simulink model "testGauges"  (R2020b)
settings: Solver=VariableStepAuto  StartTime=0.0  StopTime=10.0  RelTol=1e-3
settings Model: EnablePacing=on  VariantFading=off  Creator=grouleau  LastModifiedBy=guy

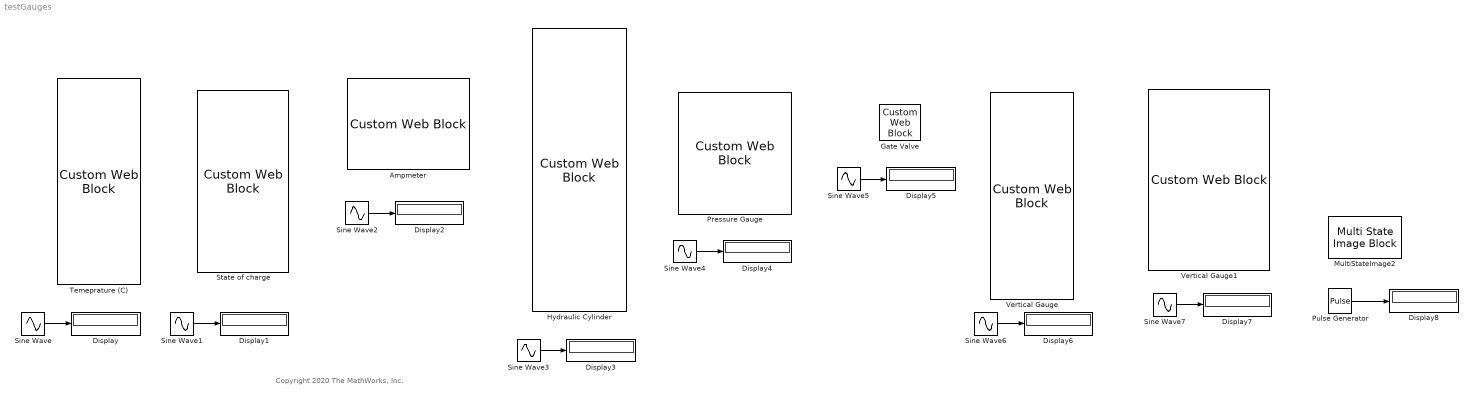
== system testGauges ==
  note: Copyright 2020 The MathWorks, Inc.
  Ampmeter : CustomWebBlock  LabelPosition=Hide  Configuration="{\"components\":[{\"name\":\"CircularScaleComponent\",\"settings\":{\"bounds\":{\"max\":12,\"min\":-12,\"tickInterval\":23.9999999999999},\"direction\":\"cw\",\"flipLimits\":0,\"innerRadius\":0.75,\"internalTickHeightScaleFactor\":1,\"labelColor\":[38,38,38],\"labelFont\":{\"font\":\"Arial\",\"fontSize\":12},\"labelTransparency\":0,\"minorTickHeightScaleFactor\":0.2,\"needleImage\":{\"size\":[96,288],\"src\":\"data:image\\/svg+xml;base64,PHN2ZyB3aWR0aD0iOTYiIGhlaWdodD0iMjg4IiB4bWxucz0iaHR0cDovL3d3dy53My5vcmcvMjAwMC9zdmciIHhtbG5zOnhsaW5rPSJodHRwOi8vd3d3LnczLm9yZy8xOTk5L3hsaW5rIiBvdmVyZmxvdz0iaGlkZGVuIj48ZGVmcz48Y2xpcFBhdGggaWQ9ImNsaXAwIj48cGF0aCBkPSJNMCAwIDk2IDAgOTYgMjg4IDAgMjg4WiIgZmlsbC1ydWxlPSJldmVub2RkIiBjbGlwLXJ1bGU9ImV2ZW5vZGQiLz48L2NsaXBQYXRoPjwvZGVmcz48ZyBjbGlwLXBhdGg9InVybCgjY2xpcDApIj48cmVjdCB4PSIwIiB5PSIwIiB3aWR0aD0iOTYiIGhlaWdodD0iMjg4IiBmaWxsPSIjRkZGRkZGIiBmaWxsLW9wYWNpdHk9IjAiLz48cGF0aCBkPSJNNDguNTAwMSA0MS41MDAxIDQ4LjUwMDIgMjQ3LjUiIHN0cm9rZT0iIzAwMDAwMCIgc3Ryb2tlLXdpZHRoPSI3IiBzdHJva2UtbGluZWNhcD0icm91bmQiIHN0cm9rZS1taXRlcmxpbWl0PSI4IiBmaWxsPSJub25lIiBmaWxsLXJ1bGU9ImV2ZW5vZGQiLz48L2c+PC9zdmc+\"},\"needleOffset\":[0.09442302068368028,0],\"needleOrientation\":-45,\"needleRotation\":90,\"needleSize\":{\"height\":0.36796446559573437,\"width\":0.26380868795837903},\"outerRadius\":0.9,\"position\":[0.17317708333333334,0.05625,0.891796875,0.7701822916666666],\"scaleAngle\":145.25613527122786,\"scaleAngleOffset\":197.0817568691423,\"scaleColors\":[],\"scaleColorsSize\":0.2,\"scalePosition\":[0,0,1,1],\"showLabels\":1,\"showMinorTicks\":1,\"showSpanLine\":1,\"showTicks\":1,\"tickColor\":[0,0,0],\"tickTransparency\":1,\"valueBarColor\":[0,114,189],\"valueBarPosition\":[0,0,1,1],\"valueBarSize\":0.2,\"valueBarTransparency\":0}},{\"name\":\"BackgroundImageComponent\",\"settings\":{\"image\":{\"size\":[384,288],\"src\":\"data:image\\/svg+xml;base64,PHN2ZyB3aWR0aD0iMzg0IiBoZWlnaHQ9IjI4OCIgeG1sbnM9Imh0dHA6Ly93d3cudzMub3JnLzIwMDAvc3ZnIiB4bWxuczp4bGluaz0iaHR0cDovL3d3dy53My5vcmcvMTk5OS94bGluayIgb3ZlcmZsb3c9ImhpZGRlbiI+PGRlZnM+PGNsaXBQYXRoIGlkPSJjbGlwMCI+PHBhdGggZD0iTTAgMCAzODQgMCAzODQgMjg4IDAgMjg4WiIgZmlsbC1ydWxlPSJldmVub2RkIiBjbGlwLXJ1bGU9ImV2ZW5vZGQiLz48L2NsaXBQYXRoPjwvZGVmcz48ZyBjbGlwLXBhdGg9InVybCgjY2xpcDApIj48cmVjdCB4PSIwIiB5PSIwIiB3aWR0aD0iMzg0IiBoZWlnaHQ9IjI4OCIgZmlsbD0iI0ZGRkZGRiIvPjxwYXRoIGQ9Ik0yNy41MDAxIDYxLjgzNDJDMjcuNTAwMSAzOS4wMDYgNDYuMDA2IDIwLjUwMDEgNjguODM0MSAyMC41MDAxTDMxNi4xNjYgMjAuNTAwMUMzMzguOTk0IDIwLjUwMDEgMzU3LjUgMzkuMDA2IDM1Ny41IDYxLjgzNDJMMzU3LjUgMjI3LjE2NkMzNTcuNSAyNDkuOTk0IDMzOC45OTQgMjY4LjUgMzE2LjE2NiAyNjguNUw2OC44MzQxIDI2OC41QzQ2LjAwNiAyNjguNSAyNy41MDAxIDI0OS45OTQgMjcuNTAwMSAyMjcuMTY2WiIgc3Ryb2tlPSIjMDAwMDAwIiBzdHJva2Utd2lkdGg9IjciIHN0cm9rZS1taXRlcmxpbWl0PSI4IiBmaWxsPSJub25lIiBmaWxsLXJ1bGU9ImV2ZW5vZGQiLz48dGV4dCBmb250LWZhbWlseT0iQXJpYWwgUm91bmRlZCBNVCxBcmlhbCBSb3VuZGVkIE1UX01TRm9udFNlcnZpY2Usc2Fucy1zZXJpZiIgZm9udC13ZWlnaHQ9IjcwMCIgZm9udC1zaXplPSI3MiIgdHJhbnNmb3JtPSJ0cmFuc2xhdGUoMTY1LjU4MyAyNTQpIj5BPC90ZXh0PjxwYXRoIGQ9Ik00OS41MDAxIDY2LjY2NzFDNDkuNTAwMSA1My4zMiA2MC4zMiA0Mi41MDAxIDczLjY2NzEgNDIuNTAwMUwzMTEuMzMzIDQyLjUwMDFDMzI0LjY4IDQyLjUwMDEgMzM1LjUgNTMuMzIgMzM1LjUgNjYuNjY3MUwzMzUuNSAxNjMuMzMzQzMzNS41IDE3Ni42OCAzMjQuNjggMTg3LjUgMzExLjMzMyAxODcuNUw3My42NjcxIDE4Ny41QzYwLjMyIDE4Ny41IDQ5LjUwMDEgMTc2LjY4IDQ5LjUwMDEgMTYzLjMzM1oiIHN0cm9rZT0iIzAwMDAwMCIgc3Ryb2tlLXdpZHRoPSI3IiBzdHJva2UtbWl0ZXJsaW1pdD0iOCIgZmlsbD0ibm9uZSIgZmlsbC1ydWxlPSJldmVub2RkIi8+PHBhdGggZD0iTTE1My41IDE4N0MxNTMuNSAxNjUuNzM3IDE3MC43MzcgMTQ4LjUgMTkyIDE0OC41IDIxMy4yNjMgMTQ4LjUgMjMwLjUgMTY1LjczNyAyMzAuNSAxODcgMjMwLjUgMTg3LjExNSAyMzAuNSAxODcuMjMgMjMwLjQ5OCAxODcuMzQ2TDE5MiAxODdaIiBzdHJva2U9IiMwMDAwMDAiIHN0cm9rZS13aWR0aD0iNyIgc3Ryb2tlLW1pdGVybGltaXQ9IjgiIGZpbGw9Im5vbmUiIGZpbGwtcnVsZT0iZXZlbm9kZCIvPjwvZz48L3N2Zz4=\",\"srcOrientation\":\"horizontal\"},\"position\":[0,0,1,1],\"scaleMode\":\"0\"}},{\"name\":\"ForegroundImageComponent\",\"settings\":{\"image\":{\"size\":[0,0],\"src\":\"default\",\"srcOrientation\":[]},\"isForeground\":1,\"position\":[0,0,1,1],\"scaleMode\":\"0\"}}],\"settings\":{\"BindingType\":\"signal\",\"aspectRatio\":1.3333333333333333,\"direction\":\"cw\",\"fixedAspectRatio\":\"on\",\"flipLimits\":0,\"orientation\":\"horizontal\",\"value\":-12},\"type\":\"CircularGauge\"}"
  Display{,1..8} (9 alike) : Display
  Gate Valve : CustomWebBlock  LabelPosition=Hide  Configuration="{\"components\":[{\"name\":\"LinearScaleComponent\",\"settings\":{\"bounds\":{\"max\":1,\"min\":0,\"tickInterval\":\"auto\"},\"internalTickHeightScaleFactor\":0.5,\"labelColor\":[250,245,199],\"labelFont\":{\"font\":\"Arial\",\"fontSize\":12},\"labelTransparency\":0,\"needleImage\":{\"size\":[0,0],\"src\":\"\",\"srcOrientation\":\"vertical\"},\"needleOffset\":[0,0],\"needleSize\":{\"height\":0,\"width\":0},\"position\":[0.036458333333333336,0.0695754716981132,3.4033018867924527,0.919921875],\"scaleColors\":[],\"scaleColorsSize\":0.2,\"showLabels\":1,\"showMinorTicks\":0,\"showSpanLine\":1,\"showTicks\":1,\"tickColor\":[250,245,200],\"tickTransparency\":0,\"valueBarColor\":[0,0,0],\"valueBarOffset\":0,\"valueBarSize\":0.23,\"valueBarTransparency\":1}},{\"name\":\"BackgroundImageComponent\",\"settings\":{\"image\":{\"size\":[0,0],\"src\":\"default\",\"srcOrientation\":null},\"position\":[0,0,1,1],\"scaleMode\":\"0\"}},{\"name\":\"ForegroundImageComponent\",\"settings\":{\"image\":{\"size\":[53,48],\"src\":\"data:image\\/png;base64,iVBORw0KGgoAAAANSUhEUgAAAp0AAAJbCAYAAACmZC+XAAAACXBIWXMAAA7EAAAOxAGVKw4bAAAAB3RJTUUH5AoDETghXxYhmQAAIABJREFUeJzs3XtwVeW9\\/\\/HPLqBEKwRNuA3BpAoElJsBArEmgtwsRUkEWqiECug0iMgPM8Fr05wZR0+agwoRLEoqwRJFIKnIMQGEBksgQORmuWMiMFwEJWBruMX1+4OSAzZr7Z2w98rea79fM4xOnmctvtOa\\/Xz291kXl2EYhgAAAAAf+klDFwAAAADnI3QCAADA5widAAAA8DlCJwAAAHyO0AkAAACfI3QCAADA5widAAAA8DlCJwAAAHyu8fUc7HK5vFUHAAAAAkR93i1EpxMAAAA+R+gEAACAzx ...(+27118 chars)\",\"srcOrientation\":\"vertical\"},\"isForeground\":1,\"position\":[0,0,1,1],\"scaleMode\":\"0\"}}],\"settings\":{\"BindingType\":\"signal\",\"aspectRatio\":0.2647058823529412,\"fixedAspectRatio\":\"off\",\"orientation\":\"vertical\",\"value\":0},\"type\":\"LinearGauge\"}"
  Hydraulic Cylinder : CustomWebBlock  LabelPosition=Hide  Configuration="{\"components\":[{\"name\":\"LinearScaleComponent\",\"settings\":{\"bounds\":{\"max\":12,\"min\":0,\"tickInterval\":\"auto\"},\"internalTickHeightScaleFactor\":0.5,\"labelColor\":[250,245,199],\"labelFont\":{\"font\":\"Arial\",\"fontSize\":12},\"labelTransparency\":0,\"needleImage\":{\"size\":[192,576],\"src\":\"data:image\\/svg+xml;base64,PHN2ZyB3aWR0aD0iMTkyIiBoZWlnaHQ9IjU3NiIgeG1sbnM9Imh0dHA6Ly93d3cudzMub3JnLzIwMDAvc3ZnIiB4bWxuczp4bGluaz0iaHR0cDovL3d3dy53My5vcmcvMTk5OS94bGluayIgb3ZlcmZsb3c9ImhpZGRlbiI+PGRlZnM+PGNsaXBQYXRoIGlkPSJjbGlwMCI+PHBhdGggZD0iTTAgMCAxOTIgMCAxOTIgNTc2IDAgNTc2WiIgZmlsbC1ydWxlPSJldmVub2RkIiBjbGlwLXJ1bGU9ImV2ZW5vZGQiLz48L2NsaXBQYXRoPjwvZGVmcz48ZyBjbGlwLXBhdGg9InVybCgjY2xpcDApIj48cmVjdCB4PSIwIiB5PSIwIiB3aWR0aD0iMTkyIiBoZWlnaHQ9IjU3NiIgZmlsbD0iI0ZGRkZGRiIgZmlsbC1vcGFjaXR5PSIwIi8+PHJlY3QgeD0iNzkuNTAwMSIgeT0iMTIxLjUiIHdpZHRoPSIzMiIgaGVpZ2h0PSI0NTIiIHN0cm9rZT0iIzAwMDAwMCIgc3Ryb2tlLXdpZHRoPSI3IiBzdHJva2UtbWl0ZXJsaW1pdD0iOCIgZmlsbD0iI0E2QTZBNiIvPjxwYXRoIGQ9Ik00MC41MDAxIDU4QzQwLjUwMDEgMjcuOTAwNSA2NC45MDA1IDMuNTAwMDUgOTUgMy41MDAwNSAxMjUuMSAzLjUwMDA1IDE0OS41IDI3LjkwMDUgMTQ5LjUgNTggMTQ5LjUgODguMDk5NiAxMjUuMSAxMTIuNSA5NSAxMTIuNSA2NC45MDA1IDExMi41IDQwLjUwMDEgODguMDk5NiA0MC41MDAxIDU4WiIgc3Ryb2tlPSIjMDAwMDAwIiBzdHJva2Utd2lkdGg9IjUiIHN0cm9rZS1taXRlcmxpbWl0PSI4IiBmaWxsPSIjNDQ3MkM0IiBmaWxsLXJ1bGU9ImV2ZW5vZGQiLz48cmVjdCB4PSI2MS41MDAxIiB5PSIxMDEuNSIgd2lkdGg9IjY5IiBoZWlnaHQ9IjIwIiBzdHJva2U9IiMwMDAwMDAiIHN0cm9rZS13aWR0aD0iNyIgc3Ryb2tlLW1pdGVybGltaXQ9IjgiIGZpbGw9IiM0NDcyQzQiLz48cGF0aCBkPSJNNjQuNTAwMSA1NS4wMDAxQzY0LjUwMDEgMzguMTU1NCA3OC4xNTU0IDI0LjUwMDEgOTUuMDAwMSAyNC41MDAxIDExMS44NDUgMjQuNTAwMSAxMjUuNSAzOC4xNTU0IDEyNS41IDU1LjAwMDEgMTI1LjUgNzEuODQ0NyAxMTEuODQ1IDg1LjUwMDEgOTUuMDAwMSA4NS41MDAxIDc4LjE1NTQgODUuNTAwMSA2NC41MDAxIDcxLjg0NDcgNjQuNTAwMSA1NS4wMDAxWiIgc3Ryb2tlPSIjMDAwMDAwIiBzdHJva2Utd2lkdGg9IjUiIHN0cm9rZS1taXRlcmxpbWl0PSI4IiBmaWxsPSIjRkZGRkZGIiBmaWxsLXJ1bGU9ImV2ZW5vZGQiLz48L2c+PC9zdmc+\",\"srcOrientation\":\"vertical\"},\"needleOffset\":[0.1248509420462676,-0.19590382902938558],\"needleSize\":{\"height\":0.5599626068376068,\"width\":0.5998931623931624},\"position\":[0.2412014563106796,0.2516084558823529,0.5994944852941176,0.39638956310679613],\"scaleColors\":[],\"scaleColorsSize\":0.2,\"showLabels\":1,\"showMinorTicks\":0,\"showSpanLine\":1,\"showTicks\":1,\"tickColor\":[250,245,200],\"tickTransparency\":0,\"valueBarColor\":[23,89,176],\"valueBarOffset\":0,\"valueBarSize\":0.23,\"valueBarTransparency\":0}},{\"name\":\"BackgroundImageComponent\",\"settings\":{\"image\":{\"size\":[0,0],\"src\":\"default\",\"srcOrientation\":null},\"position\":[0,0,1,1],\"scaleMode\":\"0\"}},{\"name\":\"ForegroundImageComponent\",\"settings\":{\"image\":{\"size\":[288,1056],\"src\":\"data:image\\/svg+xml;base64,PHN2ZyB3aWR0aD0iMjg4IiBoZWlnaHQ9IjEwNTYiIHhtbG5zPSJodHRwOi8vd3d3LnczLm9yZy8yMDAwL3N2ZyIgeG1sbnM6eGxpbms9Imh0dHA6Ly93d3cudzMub3JnLzE5OTkveGxpbmsiIG92ZXJmbG93PSJoaWRkZW4iPjxkZWZzPjxjbGlwUGF0aCBpZD0iY2xpcDAiPjxwYXRoIGQ9Ik0wIDAgMjg4IDAgMjg4IDEwNTYgMCAxMDU2WiIgZmlsbC1ydWxlPSJldmVub2RkIiBjbGlwLXJ1bGU9ImV2ZW5vZGQiLz48L2NsaXBQYXRoPjwvZGVmcz48ZyBjbGlwLXBhdGg9InVybCgjY2xpcDApIj48cmVjdCB4PSIwIiB5PSIwIiB3aWR0aD0iMjg4IiBoZWlnaHQ9IjEwNTYiIGZpbGw9IiNGRkZGRkYiIGZpbGwtb3BhY2l0eT0iMCIvPjxyZWN0IHg9Ijg1LjUwMDEiIHk9IjYzMC41IiB3aWR0aD0iMTE1IiBoZWlnaHQ9IjM2NyIgc3Ryb2tlPSIjMDAwMDAwIiBzdHJva2Utd2lkdGg9IjciIHN0cm9rZS1taXRlcmxpbWl0PSI4IiBmaWxsPSIjNDQ3MkM0Ii8+PHJlY3QgeD0iNzEuNTAwMSIgeT0iNTgxLjUiIHdpZHRoPSIxNDYiIGhlaWdodD0iNDkiIHN0cm9rZT0iIzAwMDAwMCIgc3Ryb2tlLXdpZHRoPSI3IiBzdHJva2UtbWl0ZXJsaW1pdD0iOCIgZmlsbD0iIzQ0NzJDNCIvPjxwYXRoIGQ9Ik0yMDAuNSA5ODkuNUMyMDAuNSAxMDIxLjUzIDE3NC43NTYgMTA0Ny41IDE0MyAxMDQ3LjUgMTExLjQ5IDEwNDcuNSA4NS44NTAyIDEwMjEuOTIgODUuNTAzNCA5OTAuMTM4TDE0MyA5ODkuNVoiIHN0cm9rZT0iIzAwMDAwMCIgc3Ryb2tlLXdpZHRoPSI3IiBzdHJva2UtbWl0ZXJsaW1pdD0iOCIgZmlsbD0iIzQ0NzJDNCIgZmlsbC1ydWxlPSJldmVub2RkIi8+PHJlY3QgeD0iOTAiIHk9Ijk0NSIgd2lkdGg9IjEwOCIgaGVpZ2h0PSI0OSIgZmlsbD0iIzQ0NzJDNCIvPjxwYXRoIGQ9Ik0xMDguNSA5ODkuNUMxMDguNSA5NjkuNjE4IDEyNC42MTggOTUzLjUgMTQ0LjUgOTUzLjUgMTY0LjM4MiA5NTMuNSAxODAuNSA5NjkuNjE4IDE4MC41IDk4OS41IDE4MC41IDEwMDkuMzggMTY0LjM4MiAxMDI1LjUgMTQ0LjUgMTAyNS41IDEyNC42MTggMTAyNS41IDEwOC41IDEwMDkuMzggMTA4LjUgOTg5LjVaIiBzdHJva2U9IiMwMDAwMDAiIHN0cm9rZS13aWR0aD0iNSIgc3Ryb2tlLW1pdGVybGltaXQ9IjgiIGZpbGw9IiNGRkZGRkYiIGZpbGwtcnVsZT0iZXZlbm9kZCIvPjwvZz48L3N2Zz4=\",\"srcOrientation\":\"vertical\"},\"isForeground\":1,\"position\":[0,0,1,1],\"scaleMode\":\"0\"}}],\"settings\":{\"BindingType\":\"signal\",\"aspectRatio\":0.3333333333333333,\"fixedAspectRatio\":\"on\",\"orientation\":\"vertical\",\"value\":0},\"type\":\"LinearGauge\"}"
  MultiStateImage2 : MultiStateImageBlock  LabelPosition=Hide
  Pressure Gauge : CustomWebBlock  LabelPosition=Hide  Configuration="{\"components\":[{\"name\":\"CircularScaleComponent\",\"settings\":{\"bounds\":{\"max\":2500,\"min\":0,\"tickInterval\":\"auto\"},\"direction\":\"cw\",\"flipLimits\":0,\"innerRadius\":0.75,\"internalTickHeightScaleFactor\":1,\"labelColor\":[38,38,38],\"labelFont\":{\"font\":\"Arial\",\"fontSize\":12},\"labelTransparency\":1,\"minorTickHeightScaleFactor\":0.2,\"needleImage\":{\"size\":[79,20],\"src\":\"data:image\\/svg+xml;base64,PD94bWwgdmVyc2lvbj0iMS4wIiBlbmNvZGluZz0idXRmLTgiPz4KPCEtLSBHZW5lcmF0b3I6IEFkb2JlIElsbHVzdHJhdG9yIDI0LjEuMiwgU1ZHIEV4cG9ydCBQbHVnLUluIC4gU1ZHIFZlcnNpb246IDYuMDAgQnVpbGQgMCkgIC0tPgo8c3ZnIHZlcnNpb249IjEuMSIgaWQ9IkxheWVyXzEiIHhtbG5zPSJodHRwOi8vd3d3LnczLm9yZy8yMDAwL3N2ZyIgeG1sbnM6eGxpbms9Imh0dHA6Ly93d3cudzMub3JnLzE5OTkveGxpbmsiIHg9IjBweCIgeT0iMHB4IgoJIHZpZXdCb3g9IjAgMCA3OC43IDIwIiBzdHlsZT0iZW5hYmxlLWJhY2tncm91bmQ6bmV3IDAgMCA3OC43IDIwOyIgeG1sOnNwYWNlPSJwcmVzZXJ2ZSI+CjxwYXRoIGQ9Ik01My4xLDUuOGwyNS42LTEuNGwtMy41LDVsMy4xLDUuMmwtMjUuNC0xLjNjLTEuNSwyLjMtNC4yLDMuNC02LjksM2MtMi4yLTAuMy00LjItMS43LTUuMi0zLjdMMC45LDEwLjgKCWMtMS4xLDAtMS4yLTEuNi0wLjEtMS43bDM5LjktMi43QzQyLDMuNiw0NSwyLDQ4LDIuNEM1MC4yLDIuOCw1Miw0LDUzLjEsNS44TDUzLjEsNS44eiBNNTMuNywxMS42bDIxLjQsMS4xbC0yLTMuNGwyLjEtMy4xCglMNTMuOCw3LjVDNTMuOSw4LDU0LDguNSw1NCw5LjFDNTQuMSw5LjksNTQsMTAuOCw1My43LDExLjZMNTMuNywxMS42eiBNNDAuMSw4LjJMMTkuMyw5LjVjLTMuOSwwLjMtMy45LDAuMiwwLDAuNGwyMC45LDEKCUM0MCwxMC41LDQwLDEwLDQwLDkuNUM0MCw5LjEsNDAsOC42LDQwLjEsOC4yTDQwLjEsOC4yeiBNNDcuOCw0LjFjLTMuMy0wLjUtNi4yLDIuMS02LjEsNS40YzAsMi42LDEuOSw0LjgsNC41LDUuMQoJYzMuMywwLjUsNi4zLTIuMiw2LjEtNS41QzUyLjIsNi42LDUwLjMsNC41LDQ3LjgsNC4xTDQ3LjgsNC4xeiIvPgo8L3N2Zz4K\"},\"needleOffset\":[0.061149395709068396,0],\"needleOrientation\":-45,\"needleRotation\":180,\"needleSize\":{\"height\":0.1101177838554453,\"width\":0.43719941652583294},\"outerRadius\":0.9,\"position\":[0.0065,0.1379808323486937,0.7195746356833399,0.726],\"scaleAngle\":270,\"scaleAngleOffset\":135,\"scaleColors\":[],\"scaleColorsSize\":0.2,\"scalePosition\":[0,0,1,1],\"showLabels\":1,\"showMinorTicks\":1,\"showSpanLine\":1,\"showTicks\":1,\"tickColor\":[38,38,38],\"tickTransparency\":1,\"valueBarColor\":[0,114,189],\"valueBarPosition\":[0,0,1,1],\"valueBarSize\":0.2,\"valueBarTransparency\":0}},{\"name\":\"BackgroundImageComponent\",\"settings\":{\"image\":{\"size\":[6248,6456],\"src\":\"data:image\\/svg+xml;base64,PD94bWwgdmVyc2lvbj0iMS4wIiBlbmNvZGluZz0idXRmLTgiPz4KPCEtLSBHZW5lcmF0b3I6IEFkb2JlIElsbHVzdHJhdG9yIDI0LjEuMiwgU1ZHIEV4cG9ydCBQbHVnLUluIC4gU1ZHIFZlcnNpb246IDYuMDAgQnVpbGQgMCkgIC0tPgo8c3ZnIHZlcnNpb249IjEuMSIgaWQ9IkxheWVyXzEiIHhtbG5zOnhvZG09Imh0dHA6Ly93d3cuY29yZWwuY29tL2NvcmVsZHJhdy9vZG0vMjAwMyIKCSB4bWxucz0iaHR0cDovL3d3dy53My5vcmcvMjAwMC9zdmciIHhtbG5zOnhsaW5rPSJodHRwOi8vd3d3LnczLm9yZy8xOTk5L3hsaW5rIiB4 ...(+3504 chars)\",\"srcOrientation\":\"horizontal\"},\"position\":[0,0,1,1],\"scaleMode\":\"0\"}},{\"name\":\"ForegroundImageComponent\",\"settings\":{\"image\":{\"size\":[0,0],\"src\":\"default\",\"srcOrientation\":[]},\"isForeground\":1,\"position\":[0,0,1,1],\"scaleMode\":\"0\"}}],\"settings\":{\"BindingType\":\"signal\",\"aspectRatio\":0.9677819083023544,\"direction\":\"cw\",\"fixedAspectRatio\":\"on\",\"flipLimits\":0,\"orientation\":\"horizontal\",\"value\":0},\"type\":\"CircularGauge\"}"
  Pulse Generator : DiscretePulseGenerator  PulseType=Time based  Period=4  PulseWidth=50
  Sine Wave : Sin  Amplitude=25  Bias=25  SampleTime=0
  Sine Wave1 : Sin  Amplitude=0.5  Bias=0.5  SampleTime=0
  Sine Wave2 : Sin  Amplitude=12  SampleTime=0
  Sine Wave3 : Sin  Amplitude=6  Bias=6  SampleTime=0
  Sine Wave4 : Sin  Amplitude=2500/2  Bias=2500/2  SampleTime=0
  Sine Wave5 : Sin  Amplitude=0.5  Bias=0.5  SampleTime=0
  Sine Wave6 : Sin  Amplitude=12.5  Bias=12.5  SampleTime=0
  Sine Wave7 : Sin  Amplitude=50  Bias=50  SampleTime=0
  State of charge : CustomWebBlock  LabelPosition=Hide  Configuration="{\"components\":[{\"name\":\"LinearScaleComponent\",\"settings\":{\"bounds\":{\"max\":1,\"min\":0,\"tickInterval\":0.2},\"internalTickHeightScaleFactor\":0.5,\"labelColor\":[0,0,0],\"labelFont\":{\"font\":\"Arial\",\"fontSize\":12},\"labelTransparency\":0,\"needleImage\":{\"size\":[0,0],\"src\":\"\",\"srcOrientation\":\"vertical\"},\"needleOffset\":[0,0],\"needleSize\":{\"height\":0,\"width\":0},\"position\":[0.0662421218487395,0.10333508403361344,2.7942489495798317,0.9641544117647058],\"scaleColors\":[],\"scaleColorsSize\":0.2,\"showLabels\":1,\"showMinorTicks\":0,\"showSpanLine\":1,\"showTicks\":1,\"tickColor\":[38,38,38],\"tickTransparency\":0,\"valueBarColor\":[23,89,176],\"valueBarOffset\":0,\"valueBarSize\":0.23,\"valueBarTransparency\":1}},{\"name\":\"BackgroundImageComponent\",\"settings\":{\"image\":{\"size\":[192,384],\"src\":\"data:image\\/svg+xml;base64,PHN2ZyB3aWR0aD0iMTkyIiBoZWlnaHQ9IjM4NCIgeG1sbnM9Imh0dHA6Ly93d3cudzMub3JnLzIwMDAvc3ZnIiB4bWxuczp4bGluaz0iaHR0cDovL3d3dy53My5vcmcvMTk5OS94bGluayIgb3ZlcmZsb3c9ImhpZGRlbiI+PGRlZnM+PGNsaXBQYXRoIGlkPSJjbGlwMCI+PHBhdGggZD0iTTAgMCAxOTIgMCAxOTIgMzg0IDAgMzg0WiIgZmlsbC1ydWxlPSJldmVub2RkIiBjbGlwLXJ1bGU9ImV2ZW5vZGQiLz48L2NsaXBQYXRoPjwvZGVmcz48ZyBjbGlwLXBhdGg9InVybCgjY2xpcDApIj48cmVjdCB4PSIwIiB5PSIwIiB3aWR0aD0iMTkyIiBoZWlnaHQ9IjM4NCIgZmlsbD0iI0ZGRkZGRiIvPjxwYXRoIGQ9Ik0yMi41MDAxIDU4LjUwMDVDMjIuNTAwMSA0NC42OTMxIDMzLjY5MzEgMzMuNTAwMSA0Ny41MDA1IDMzLjUwMDFMMTQ3LjUgMzMuNTAwMUMxNjEuMzA3IDMzLjUwMDEgMTcyLjUgNDQuNjkzMSAxNzIuNSA1OC41MDA1TDE3Mi41IDM1My41QzE3Mi41IDM2Ny4zMDcgMTYxLjMwNyAzNzguNSAxNDcuNSAzNzguNUw0Ny41MDA1IDM3OC41QzMzLjY5MzEgMzc4LjUgMjIuNTAwMSAzNjcuMzA3IDIyLjUwMDEgMzUzLjVaIiBzdHJva2U9IiMwMDAwMDAiIHN0cm9rZS13aWR0aD0iNyIgc3Ryb2tlLW1pdGVybGltaXQ9IjgiIGZpbGw9Im5vbmUiIGZpbGwtcnVsZT0iZXZlbm9kZCIvPjxwYXRoIGQ9Ik01NiA4LjAwMDA5QzU2IDUuMjM4NjIgNTguMjM4NiAzIDYxLjAwMDEgM0wxMzMgM0MxMzUuNzYxIDMgMTM4IDUuMjM4NjIgMTM4IDguMDAwMDlMMTM4IDI3Ljk5OTlDMTM4IDMwLjc2MTQgMTM1Ljc2MSAzMyAxMzMgMzNMNjEuMDAwMSAzM0M1OC4yMzg2IDMzIDU2IDMwLjc2MTQgNTYgMjcuOTk5OVoiIGZpbGwtcnVsZT0iZXZlbm9kZCIvPjwvZz48L3N2Zz4=\",\"srcOrientation\":\"vertical\"},\"position\":[0,0,1,1],\"scaleMode\":\"0\"}},{\"name\":\"ForegroundImageComponent\",\"settings\":{\"image\":{\"size\":[0,0],\"src\":\"default\",\"srcOrientation\":[]},\"isForeground\":1,\"position\":[0,0,1,1],\"scaleMode\":\"0\"}}],\"settings\":{\"BindingType\":\"signal\",\"aspectRatio\":0.5,\"fixedAspectRatio\":\"on\",\"orientation\":\"vertical\"},\"type\":\"LinearGauge\"}"
  Temeprature (C) : CustomWebBlock  LabelPosition=Hide  Configuration="{\"components\":[{\"name\":\"LinearScaleComponent\",\"settings\":{\"bounds\":{\"max\":50,\"min\":0,\"tickInterval\":\"auto\"},\"internalTickHeightScaleFactor\":0.5,\"labelColor\":[38,38,38],\"labelFont\":{\"font\":\"Arial\",\"fontSize\":12},\"labelTransparency\":1,\"needleImage\":{\"size\":[0,0],\"src\":\"\",\"srcOrientation\":\"vertical\"},\"needleOffset\":[0,0],\"needleSize\":{\"height\":0,\"width\":0},\"position\":[0.06567112546125461,0.0888569374550683,1.3367361610352264,0.692054889298893],\"scaleColors\":[],\"scaleColorsSize\":0.2,\"showLabels\":1,\"showMinorTicks\":0,\"showSpanLine\":1,\"showTicks\":1,\"tickColor\":[0,0,0],\"tickTransparency\":0,\"valueBarColor\":[194,0,0],\"valueBarOffset\":0,\"valueBarSize\":0.23,\"valueBarTransparency\":1}},{\"name\":\"BackgroundImageComponent\",\"settings\":{\"image\":{\"size\":[154,384],\"src\":\"data:image\\/svg+xml;base64,PHN2ZyB3aWR0aD0iMTU0IiBoZWlnaHQ9IjM4NCIgeG1sbnM9Imh0dHA6Ly93d3cudzMub3JnLzIwMDAvc3ZnIiB4bWxuczp4bGluaz0iaHR0cDovL3d3dy53My5vcmcvMTk5OS94bGluayIgb3ZlcmZsb3c9ImhpZGRlbiI+PGRlZnM+PGNsaXBQYXRoIGlkPSJjbGlwMCI+PHBhdGggZD0iTTAgMCAxNTQgMCAxNTQgMzg0IDAgMzg0WiIgZmlsbC1ydWxlPSJldmVub2RkIiBjbGlwLXJ1bGU9ImV2ZW5vZGQiLz48L2NsaXBQYXRoPjwvZGVmcz48ZyBjbGlwLXBhdGg9InVybCgjY2xpcDApIj48cmVjdCB4PSIwIiB5PSIwIiB3aWR0aD0i ...(+1892 chars)\",\"srcOrientation\":\"vertical\"},\"position\":[0,0,1,1],\"scaleMode\":\"0\"}},{\"name\":\"ForegroundImageComponent\",\"settings\":{\"image\":{\"size\":[0,0],\"src\":\"default\",\"srcOrientation\":[]},\"isForeground\":1,\"position\":[0,0,1,1],\"scaleMode\":\"0\"}}],\"settings\":{\"BindingType\":\"signal\",\"aspectRatio\":0.4010416666666667,\"fixedAspectRatio\":\"on\",\"orientation\":\"vertical\"},\"type\":\"LinearGauge\"}"
  Vertical Gauge : CustomWebBlock  LabelPosition=Hide  ShowInitialText=on  Configuration="{\"components\":[{\"name\":\"LinearScaleComponent\",\"settings\":{\"bounds\":{\"max\":25,\"min\":0,\"tickInterval\":\"auto\"},\"internalTickHeightScaleFactor\":1,\"labelColor\":[38,38,38],\"labelFont\":{\"font\":\"Arial\",\"fontSize\":12},\"labelTransparency\":1,\"needleImage\":{\"size\":[298,298],\"src\":\"data:image\\/svg+xml;base64,PHN2ZyB3aWR0aD0iMjk4IiBoZWlnaHQ9IjI5OCIgeG1sbnM9Imh0dHA6Ly93d3cudzMub3JnLzIwMDAvc3ZnIiB4bWxuczp4bGluaz0iaHR0cDovL3d3dy53My5vcmcvMTk5OS94bGluayIgb3ZlcmZsb3c9ImhpZGRlbiI+PGRlZnM+PGNsaXBQYXRoIGlkPSJjbGlwMCI+PHBhdGggZD0iTTAgMCAyOTggMCAyOTggMjk4IDAgMjk4WiIgZmlsbC1ydWxlPSJldmVub2RkIiBjbGlwLXJ1bGU9ImV2ZW5vZGQiLz48L2NsaXBQYXRoPjxyYWRpYWxHcmFkaWVudCBjeD0iMS4wNjU2MWUrMDYiIGN5PSIxLjA2NTYxZSswNiIgcj0iMS41MDdlKzA2IiBmeD0iMS4wNjU2MWUrMDYiIGZ5PSIxLjA2NTYxZSswNiIgZ3JhZGllbnRVbml0cz0idXNlclNwYWNlT25Vc2UiIHNwcmVhZE1ldGhvZD0icGFkIiBpZD0iZmlsbDEiIGdyYWRpZW50VHJhbnNmb3JtPSJtYXRyaXgoMC4wMDAxMDUxMDQgMCAwIDAuMDAwMTA1MTA0IDM3IDQ5KSI+PHN0b3Agb2Zmc2V0PSIwIiBzdG9wLWNvbG9yPSIjQjA1MDBGIi8+PHN0b3Agb2Zmc2V0PSIwLjQ4IiBzdG9wLWNvbG9yPSIjRUU4MTM3Ii8+PHN0b3Agb2Zmc2V0PSIxIiBzdG9wLWNvbG9yPSIjRjRCMTgzIi8+PC9yYWRpYWxHcmFkaWVudD48L2RlZnM+PGcgY2xpcC1wYXRoPSJ1cmwoI2NsaXAwKSI+PHJlY3QgeD0iMCIgeT0iMCIgd2lkdGg9IjI5OCIgaGVpZ2h0PSIyOTgiIGZpbGw9IiNGRkZGRkYiIGZpbGwtb3BhY2l0eT0iMCIvPjxwYXRoIGQ9Ik0zNyAxNjFDMzcgOTkuMTQ0MSA4Ny4xNDQxIDQ5IDE0OSA0OSAyMTAuODU2IDQ5IDI2MSA5OS4xNDQxIDI2MSAxNjEgMjYxIDIyMi44NTYgMjEwLjg1NiAyNzMgMTQ5IDI3MyA4Ny4xNDQxIDI3MyAzNyAyMjIuODU2IDM3IDE2MVoiIHN0cm9rZT0iI0VEN0QzMSIgc3Ryb2tlLXdpZHRoPSIzLjk5OTk2IiBzdHJva2UtbWl0ZXJsaW1pdD0iOCIgZmlsbD0idXJsKCNmaWxsMSkiIGZpbGwtcnVsZT0iZXZlbm9kZCIvPjwvZz48L3N2Zz4=\",\"srcOrientation\":\"vertical\"},\"needleOffset\":[-0.4190231362467866,0.06580976863753213],\"needleSize\":{\"height\":0.22511574074074073,\"width\":0.5627893518518519},\"position\":[0.12858796296296296,0.008391203703703705,1.0219907407407407,0.8446180555555556],\"scaleColors\":[],\"scaleColorsSize\":0.2,\"showLabels\":1,\"showMinorTicks\":0,\"showSpanLine\":false,\"showTicks\":1,\"tickColor\":[166,166,166],\"tickTransparency\":1,\"valueBarColor\":[23,89,176],\"valueBarOffset\":0,\"valueBarSize\":0.23,\"valueBarTransparency\":0}},{\"name\":\"BackgroundImageComponent\",\"settings\":{\"image\":{\"size\":[384,960],\"src\":\"data:image\\/svg+xml;base64,PHN2ZyB3aWR0aD0iMzg0IiBoZWlnaHQ9Ijk2MCIgeG1sbnM9Imh0dHA6Ly93d3cudzMub3JnLzIwMDAvc3ZnIiB4bWxuczp4bGluaz0iaHR0cDovL3d3dy53My5vcmcvMTk5OS94bGluayIgb3ZlcmZsb3c9ImhpZGRlbiI+PGRlZnM+PGNsaXBQYXRoIGlkPSJjbGlwMCI+PHBhdGggZD0iTTAgMCAzODQgMCAzODQgOTYwIDAgOTYwWiIgZmlsbC1ydWxlPSJldmVub2RkIiBjbGlwLXJ1bGU9ImV2ZW5vZGQiLz48L2NsaXBQYXRoPjwvZGVmcz48ZyBjbGlwLXBhdGg9InVybCgjY2xpcDApIj48cmVjdCB4PSIwIiB5PSIwIiB3aWR0aD0i ...(+2956 chars)\",\"srcOrientation\":\"vertical\"},\"position\":[0,0,1,1],\"scaleMode\":\"0\"}},{\"name\":\"ForegroundImageComponent\",\"settings\":{\"image\":{\"size\":[0,0],\"src\":\"default\",\"srcOrientation\":[]},\"isForeground\":1,\"position\":[0,0,1,1],\"scaleMode\":\"0\"}}],\"settings\":{\"BindingType\":\"signal\",\"aspectRatio\":0.4,\"fixedAspectRatio\":\"on\",\"orientation\":\"vertical\",\"value\":0},\"type\":\"LinearGauge\"}"
  Vertical Gauge1 : CustomWebBlock  LabelPosition=Hide  Configuration="{\"components\":[{\"name\":\"LinearScaleComponent\",\"settings\":{\"bounds\":{\"max\":100,\"min\":0,\"tickInterval\":\"auto\"},\"internalTickHeightScaleFactor\":1,\"labelColor\":[38,38,38],\"labelFont\":{\"font\":\"Arial\",\"fontSize\":12},\"labelTransparency\":1,\"needleImage\":{\"size\":[960,384],\"src\":\"data:image\\/svg+xml;base64,PHN2ZyB3aWR0aD0iOTYwIiBoZWlnaHQ9IjM4NCIgeG1sbnM9Imh0dHA6Ly93d3cudzMub3JnLzIwMDAvc3ZnIiB4bWxuczp4bGluaz0iaHR0cDovL3d3dy53My5vcmcvMTk5OS94bGluayIgb3ZlcmZsb3c9ImhpZGRlbiI+PGRlZnM+PGNsaXBQYXRoIGlkPSJjbGlwMCI+PHBhdGggZD0iTTAgMCA5NjAgMCA5NjAgMzg0IDAgMzg0WiIgZmlsbC1ydWxlPSJldmVub2RkIiBjbGlwLXJ1bGU9ImV2ZW5vZGQiLz48L2NsaXBQYXRoPjxpbWFnZSB3aWR0aD0iNzUiIGhlaWdodD0iODQiIHhsaW5rOmhyZWY9ImRhdGE6aW1hZ2UvanBlZzti ...(+118888 chars)\",\"srcOrientation\":\"vertical\"},\"needleOffset\":[-0.3472684876748834,0.002165982672138623],\"needleSize\":{\"height\":0.3941701680672269,\"width\":0.8638960015757337},\"position\":[0.530921743697479,0.04421902698443963,0.818790624384479,0.4299501050420168],\"scaleColors\":[],\"scaleColorsSize\":0.2,\"showLabels\":false,\"showMinorTicks\":0,\"showSpanLine\":false,\"showTicks\":false,\"tickColor\":[38,38,38],\"tickTransparency\":1,\"valueBarColor\":[0,187,205],\"valueBarOffset\":0.02,\"valueBarSize\":1,\"valueBarTransparency\":1}},{\"name\":\"BackgroundImageComponent\",\"settings\":{\"image\":{\"size\":[480,720],\"src\":\"data:image\\/svg+xml;base64,PHN2ZyB3aWR0aD0iNDgwIiBoZWlnaHQ9IjcyMCIgeG1sbnM9Imh0dHA6Ly93d3cudzMub3JnLzIwMDAvc3ZnIiB4bWxuczp4bGluaz0iaHR0cDovL3d3dy53My5vcmcvMTk5OS94bGluayIgb3ZlcmZsb3c9ImhpZGRlbiI+PGRlZnM+PGNsaXBQYXRoIGlkPSJjbGlwMCI+PHBhdGggZD0iTTAgMCA0ODAgMCA0ODAgNzIwIDAgNzIwWiIgZmlsbC1ydWxlPSJldmVub2RkIiBjbGlwLXJ1bGU9ImV2ZW5vZGQiLz48L2NsaXBQYXRoPjwvZGVmcz48ZyBjbGlwLXBhdGg9InVybCgjY2xpcDApIj48cmVjdCB4PSIwIiB5PSIwIiB3aWR0aD0i ...(+1700 chars)\",\"srcOrientation\":\"vertical\"},\"position\":[0,0,1,1],\"scaleMode\":\"0\"}},{\"name\":\"ForegroundImageComponent\",\"settings\":{\"image\":{\"size\":[0,0],\"src\":\"default\",\"srcOrientation\":[]},\"isForeground\":1,\"position\":[0,0,1,1],\"scaleMode\":\"0\"}}],\"settings\":{\"BindingType\":\"signal\",\"aspectRatio\":0.6666666666666666,\"fixedAspectRatio\":\"on\",\"orientation\":\"vertical\",\"value\":0},\"type\":\"LinearGauge\"}"
  wires:
  Sine Wave/1 -> Display/1
  Sine Wave1/1 -> Display1/1
  Sine Wave2/1 -> Display2/1
  Sine Wave3/1 -> Display3/1
  Sine Wave4/1 -> Display4/1
  Sine Wave5/1 -> Display5/1
  Sine Wave6/1 -> Display6/1
  Sine Wave7/1 -> Display7/1
  Pulse Generator/1 -> Display8/1
